simulink model "Attitude_velocity_controller"  (R2019b)
settings: Solver=ode3  StartTime=0  StopTime=9  FixedStep=0.0001  RelTol=1e-3
PreLoadFcn:
  | a = 10
values from neighbouring files (symbols this model uses):
  X0 = [px(1), py(1), pz(1), vx(1), vy(1), vz(1), 0, 0, 0]'    [traj_plot.m]
libraries: commchan3 x2
settings Model: Creator=Fredrik Skjernov  LastModifiedBy=oscar
settings DataIOCC: ReturnWorkspaceOutputs=off
settings DebuggingCC: PregeneratedLibrarySubsystemCodeDiagnostic=none  ArithmeticOperatorsInVariantConditions=warning
settings SFSimCC: SimUseLocalCustomCode=off  CustomCodeUndefinedFunction=UseInterfaceOnly
settings RTWCC: RTWUseLocalCustomCode=off

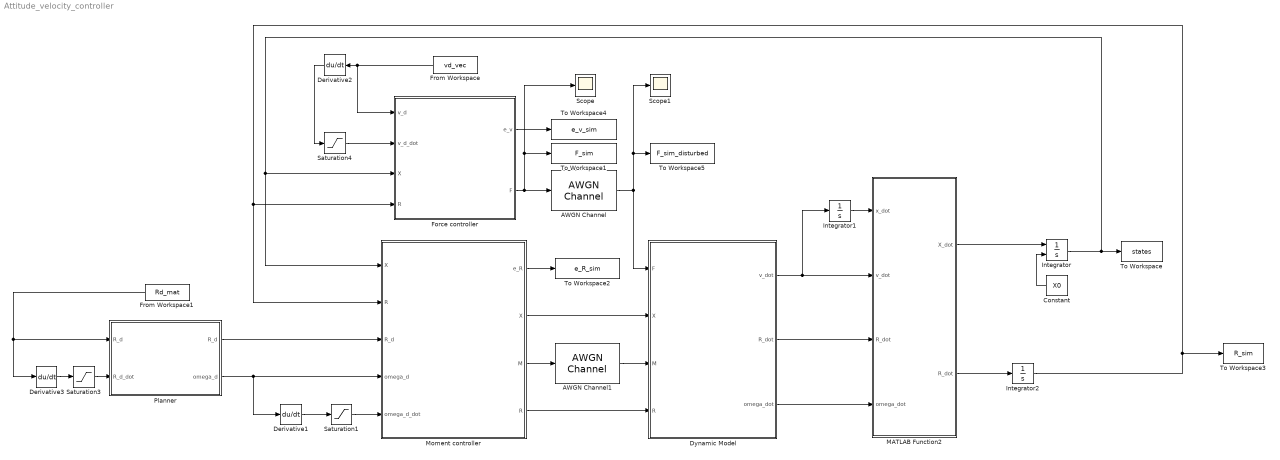
== system Attitude_velocity_controller ==
  AWGN Channel : commchan3/AWGN Channel  InputProcessing=Columns as channels (frame based)  seed=67  noiseMode="Signal to noise ratio  (Eb/No)"  EbNodB=10  EsNodB=10  SNRdB=10  bitsPerSym=1  Ps=1  Tsym=1  variance=1
      settings: SourceProductName=Communications Toolbox
  AWGN Channel1 : commchan3/AWGN Channel  InputProcessing=Columns as channels (frame based)  seed=67  noiseMode="Signal to noise ratio  (Eb/No)"  EbNodB=10  EsNodB=10  SNRdB=10  bitsPerSym=1  Ps=1  Tsym=1  variance=1
      settings: SourceProductName=Communications Toolbox
  Constant : Constant  Value=X0
  Derivative1 : Derivative
  Derivative2 : Derivative
  Derivative3 : Derivative
  Dynamic Model : MATLAB Function  TreatAsAtomicUnit=on
  Force controller : MATLAB Function  TreatAsAtomicUnit=on
  From Workspace : FromWorkspace  VariableName=vd_vec  SampleTime=0
  From Workspace1 : FromWorkspace  VariableName=Rd_mat  SampleTime=0
  Integrator : Integrator  InitialConditionSource=external  InitialCondition=[0, 0, 0, 0, 0, 0, 0, 0, 0]'
  Integrator1 : Integrator  InitialCondition=[0;0;0]
  Integrator2 : Integrator  InitialCondition=[1, 0, 0; 0, 1, 0; 0, 0, 1]
  MATLAB Function2 : MATLAB Function  TreatAsAtomicUnit=on
  Moment controller : MATLAB Function  TreatAsAtomicUnit=on
  Planner : MATLAB Function  TreatAsAtomicUnit=on
  Saturation1 : Saturate  UpperLimit=inf  LowerLimit=-inf
  Saturation3 : Saturate  UpperLimit=inf  LowerLimit=-inf
  Saturation4 : Saturate  UpperLimit=inf  LowerLimit=-inf
  Scope : Scope
  Scope1 : Scope
  To Workspace : ToWorkspace  VariableName=states  SaveFormat=Timeseries  SampleTime=-1
  To Workspace1 : ToWorkspace  VariableName=F_sim  SaveFormat=Timeseries  SampleTime=-1
  To Workspace2 : ToWorkspace  VariableName=e_R_sim  SaveFormat=Timeseries  SampleTime=-1
  To Workspace3 : ToWorkspace  VariableName=R_sim  SaveFormat=Timeseries  SampleTime=-1
  To Workspace4 : ToWorkspace  VariableName=e_v_sim  SaveFormat=Timeseries  SampleTime=-1
  To Workspace5 : ToWorkspace  VariableName=F_sim_disturbed  SaveFormat=Timeseries  SampleTime=-1
  wires:
  Moment controller/3(M) -> AWGN Channel1/1
  Dynamic Model/2(R_dot) -> MATLAB Function2/3("R_dot ")
  Dynamic Model/1(v_dot) -> Integrator1/1, MATLAB Function2/2(v_dot)
  Integrator1/1 -> MATLAB Function2/1(x_dot)
  Dynamic Model/3(omega_dot) -> MATLAB Function2/4(omega_dot)
  Moment controller/4(R) -> Dynamic Model/4(R)
  MATLAB Function2/2(R_dot) -> Integrator2/1
  Derivative3/1 -> Saturation3/1
  Planner/1(R_d) -> Moment controller/3(R_d)
  Planner/2(omega_d) -> Derivative1/1, Moment controller/4(omega_d)
  Derivative1/1 -> Saturation1/1
  Saturation1/1 -> Moment controller/5(omega_d_dot)
  MATLAB Function2/1(X_dot) -> Integrator/1
  Constant/1 -> Integrator/2
  Force controller/2(F) -> To Workspace1/1, Scope/1, AWGN Channel/1
  Derivative2/1 -> Saturation4/1
  Saturation3/1 -> Planner/2(R_d_dot)
  From Workspace1/1 -> Planner/1("R_d "), Derivative3/1
  From Workspace/1 -> Force controller/1(v_d), Derivative2/1
  Saturation4/1 -> Force controller/2(v_d_dot)
  Integrator/1 -> Moment controller/1("X "), Force controller/3(X), To Workspace/1
  Integrator2/1 -> To Workspace3/1, Moment controller/2("R "), Force controller/4(R)
  AWGN Channel/1 -> To Workspace5/1, Scope1/1, Dynamic Model/1(F)
  AWGN Channel1/1 -> Dynamic Model/3(M)
  Moment controller/2(X) -> Dynamic Model/2(X)
  Moment controller/1(e_R) -> To Workspace2/1
  Force controller/1(e_v) -> To Workspace4/1

== matlab function Attitude_velocity_controller/Dynamic Model ==
  data: v_dot output; F input; X input; M input; R_dot output; omega_dot output; R input
function [v_dot, R_dot, omega_dot]  = fcn(F,X,M, R)
omega = X(7:9);
m = 1; % massan
g = -9.81; 
% Rx = [1 0 0;0 cos(fi) -sin(fi);0 sin(fi) cos(fi)];
% Ry = [cos(theta) 0 sin(theta);0 1 0;-sin(theta) 0 cos(theta)];
% Rz = [cos(psi) -sin(psi) 0; sin(psi) cos(psi) 0; 0 0 1];
% R = Rx*Ry*Rz

e3 = [0 0 1];
J = [0.0820 0 0;0 0.0845 0;0 0 0.1377];
omega_hat = [0,-omega(3),omega(2);omega(3),0,-omega(1);-omega(2),omega(1),0];
 
R_dot = R * omega_hat;
v_dot = g*e3' + (F/m)*R*e3'; 
omega_dot = inv(J)*(M-cross(omega,J*omega));

== matlab function Attitude_velocity_controller/Planner ==
  data: R_d output; R_d input; R_d_dot input; omega_d output
function [R_d, omega_d] = fcn(R_d, R_d_dot)
omega_d_hat = R_d'*R_d_dot;
omega_d = [omega_d_hat(3,2); omega_d_hat(1,3); omega_d_hat(2,1)];

== matlab function Attitude_velocity_controller/Force controller ==
  data: e_v output; v_d input; v_d_dot input; X input; F output; R input
function [e_v, F]  = fcn(v_d, v_d_dot, X, R)
m = 1; 
g = -9.81;
k_v = 40;
e3 = [0 0 1]';
v = X(4:6);
e_v = v - v_d;
F = dot(-k_v*e_v - m*g*e3 + m*v_d_dot, R*e3);

== matlab function Attitude_velocity_controller/Moment controller ==
  data: X input; e_R output; X output; R input; R_d input; omega_d input; M output; R output; omega_d_dot input
function [e_R, X, M, R]= fcn(X, R, R_d, omega_d, omega_d_dot)
omega = X(7:9);

J = [0.0820, 0, 0;0, 0.0845, 0;0, 0, 0.1377];

k_R = 50;
k_omega = 2.5;

e_omega = omega - R'*R_d*omega_d;

e_R = (1/2).*(R_d'*R - R'*R_d);
eR_vee = [e_R(3,2);e_R(1,3);e_R(2,1)];  %inverse v-map
 
omega_hat = [0, -omega(3), omega(2); omega(3), 0, -omega(1); -omega(2), omega(1), 0];

M = -k_R*eR_vee - k_omega*e_omega + cross(omega,J*omega) - J*(omega_hat*R'*R_d*omega_d - R'*R_d*omega_d_dot);

== matlab function Attitude_velocity_controller/MATLAB Function2 ==
  data: x_dot input; v_dot input; R_dot input; omega_dot input; X_dot output; R_dot output
function [X_dot, R_dot] = fcn(x_dot, v_dot, R_dot, omega_dot)

X_dot = [x_dot; v_dot; omega_dot];
